simulink model "Tune_Abstract_BDMotor"  (R2014a)
settings: Solver=ode45  StartTime=0.0  StopTime=5  MaxStep=1e-4  RelTol=1e-3
PreLoadFcn:
  | load PQ_BDMotor_FULL
PostLoadFcn:
  | warning off Simulink:blocks:LegendInfoNA
libraries: simulink x2
Description:
  | Copyright 2014 The MathWorks, Inc.
settings Model: Creator=smiller  LastModifiedBy=psanghvi
settings DebuggingCC: UnderspecifiedInitializationDetection=Classic  StateNameClashWarn=warning

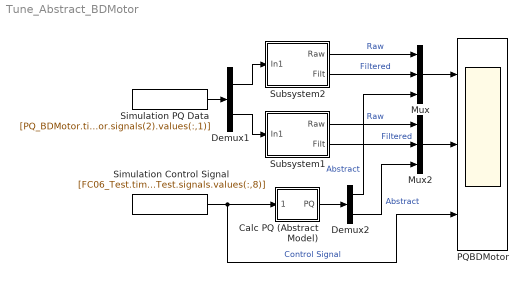
== system Tune_Abstract_BDMotor ==
  Calc PQ (Abstract Model) : Subsystem  mask{delay=5, ramp_dur=45, step_down=250, slope=792, q_scaling=0.72}
      mask prompts: delay "# Delay periods (10 ms)"; ramp_dur "# Ramp periods (10 ms)"; step_down "Peak max - steady state (W)"; slope "Ramp slope"; q_scaling "Q scale factor"
  Demux1 : Demux  Outputs=2
  Demux2 : Demux  Outputs=2
  Mux : Mux  Inputs=3
  Mux2 : Mux  Inputs=3
  PQBDMotor : Scope  NumInputPorts=3
      settings: ShowLegends=on  YMin=0~-100~-550  YMax=1500~600~550  SaveName=PQ_BDMotor  Decimation=10  SampleTime=10e-6
  Simulation Control Signal : FromWorkspace  VariableName=[FC06_Test.time FC06_Test.signals.values(:,8)]  SampleTime=0
  Simulation PQ Data : FromWorkspace  VariableName=[PQ_BDMotor.time PQ_BDMotor.signals(1).values(:,1) PQ_BDMotor.signals(2).values(:,1)]  SampleTime=0
  Subsystem1 : Subsystem
  Subsystem2 : Subsystem
  wires:
  Subsystem2/1(Raw) -> Mux/1  "Raw"
  Subsystem1/1(Raw) -> Mux2/1  "Raw"
  Simulation PQ Data/1 -> Demux1/1
  Demux1/1 -> Subsystem2/1(In1)
  Demux1/2 -> Subsystem1/1(In1)
  Simulation Control Signal/1 -> Calc PQ (Abstract Model)/1(Ctrl), PQBDMotor/3  "Control Signal"
  Calc PQ (Abstract Model)/1(PQ) -> Demux2/1
  Demux2/1 -> Mux/3  "Abstract"
  Demux2/2 -> Mux2/3  "Abstract"
  Mux/1 -> PQBDMotor/1
  Mux2/1 -> PQBDMotor/2
  Subsystem2/2(Filt) -> Mux/2  "Filtered"
  Subsystem1/2(Filt) -> Mux2/2  "Filtered"

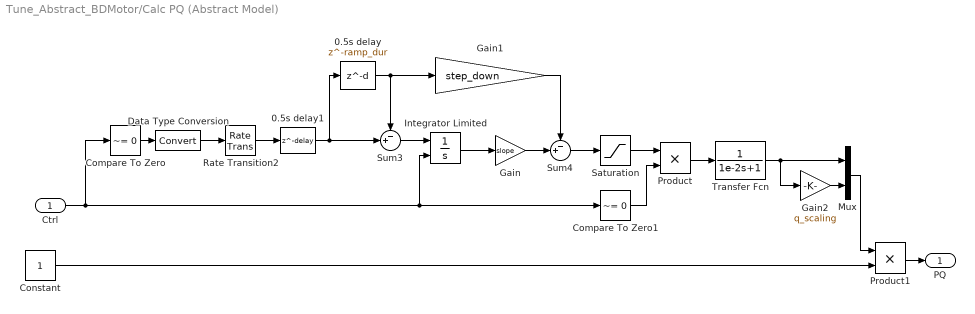
== system Tune_Abstract_BDMotor/Calc PQ (Abstract Model) ==
  Ctrl : Inport
  0.5s delay : Delay  DelayLength=ramp_dur  SampleTime=0.01
  0.5s delay1 : Delay  DelayLength=delay  SampleTime=0.01
  Compare To Zero : simulink/Logic and Bit Operations/Compare To Zero  relop=~=  OutDataTypeStr=boolean
  Compare To Zero1 : simulink/Logic and Bit Operations/Compare To Zero  relop=~=  OutDataTypeStr=boolean
  Constant : Constant
  Data Type Conversion : DataTypeConversion
  Gain : Gain  Gain=slope
  Gain1 : Gain  Gain=step_down
  Gain2 : Gain  Gain=q_scaling
  Integrator Limited : Integrator  ExternalReset=falling  LimitOutput=on  UpperSaturationLimit=1  LowerSaturationLimit=0
  Mux : Mux  Inputs=2
  Product : Product
  Product1 : Product
  Rate Transition2 : RateTransition  OutPortSampleTime=0.01
  Saturation : Saturate  UpperLimit=1160  LowerLimit=0
  Sum3 : Sum  Inputs=-+|  SaturateOnIntegerOverflow=on  InputSameDT=on  OutDataTypeStr=Inherit: Same as first input
  Sum4 : Sum  Inputs=-+|  SaturateOnIntegerOverflow=on  InputSameDT=on  OutDataTypeStr=Inherit: Same as first input
  Transfer Fcn : TransferFcn  Denominator=[1e-2 1]
  PQ : Outport
  wires:
  Product1/1 -> PQ/1
  Constant/1 -> Product1/2
  0.5s delay1/1 -> 0.5s delay/1, Sum3/2
  Ctrl/1 -> Compare To Zero/1, Compare To Zero1/1, Integrator Limited/2
  Mux/1 -> Product1/1
  Gain2/1 -> Mux/2
  Transfer Fcn/1 -> Mux/1, Gain2/1
  Compare To Zero/1 -> Data Type Conversion/1
  Integrator Limited/1 -> Gain/1
  Data Type Conversion/1 -> Rate Transition2/1
  Gain/1 -> Sum4/2
  Rate Transition2/1 -> 0.5s delay1/1
  Sum3/1 -> Integrator Limited/1
  Product/1 -> Transfer Fcn/1
  Gain1/1 -> Sum4/1
  0.5s delay/1 -> Sum3/1, Gain1/1
  Sum4/1 -> Saturation/1
  Saturation/1 -> Product/1
  Compare To Zero1/1 -> Product/2

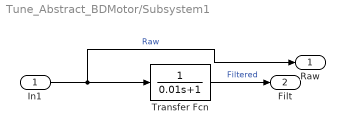
== system Tune_Abstract_BDMotor/Subsystem1 ==
  In1 : Inport
  Transfer Fcn : TransferFcn  Denominator=[0.01 1]
  Raw : Outport
  Filt : Outport  Port=2
  wires:
  In1/1 -> Transfer Fcn/1, Raw/1  "Raw"
  Transfer Fcn/1 -> Filt/1  "Filtered"

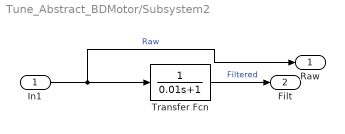
== system Tune_Abstract_BDMotor/Subsystem2 ==
  In1 : Inport
  Transfer Fcn : TransferFcn  Denominator=[0.01 1]
  Raw : Outport
  Filt : Outport  Port=2
  wires:
  Transfer Fcn/1 -> Filt/1  "Filtered"
  In1/1 -> Raw/1, Transfer Fcn/1  "Raw"
